simulink model "smart_watering_system_arduino"  (R2018b)
settings: Solver=FixedStepAuto  StartTime=0.0  StopTime=inf  RelTol=1e-3  EnableMultiTasking=on
settings Model: ExtModeTrigDuration=2  Creator=The MathWorks, Inc.  LastModifiedBy=Andrei
settings OptimizationCC: MaxStackSize=64
settings DebuggingCC: ParameterTunabilityLossMsg=error  LibraryContextMissingDiagnostic=none
settings HardwareCC: ProdBitPerInt=16  ProdBitPerPointer=16  ProdBitPerSizeT=16  ProdBitPerPtrDiffT=16  ProdLargestAtomicFloat=None  ProdWordSize=8  ProdHWDeviceType=Atmel->AVR  UseEmbeddedCoderFeatures=off  UseSimulinkCoderFeatures=off
settings SFSimCC: SimUseLocalCustomCode=off
settings RTWCC: SystemTargetFile=ert.tlc  HardwareBoard=Arduino Mega 2560  TemplateMakefile=ert_default_tmf  GenerateReport=on  RTWUseLocalCustomCode=off  Toolchain=Arduino AVR  BuildConfiguration=Faster Runs  LaunchReport=on
settings CodeAppCC: ForceParamTrailComments=on  OperatorAnnotations=on  StateflowObjectComments=on  MATLABSourceComments=on
settings ERTTargetCC: ERTCustomFileBanners=off  SupportContinuousTime=on  SupportNonInlinedSFcns=on  RemoveResetFunc=off  SupportVariableSizeSignals=on  ModelStepFunctionPrototypeControlCompliant=off

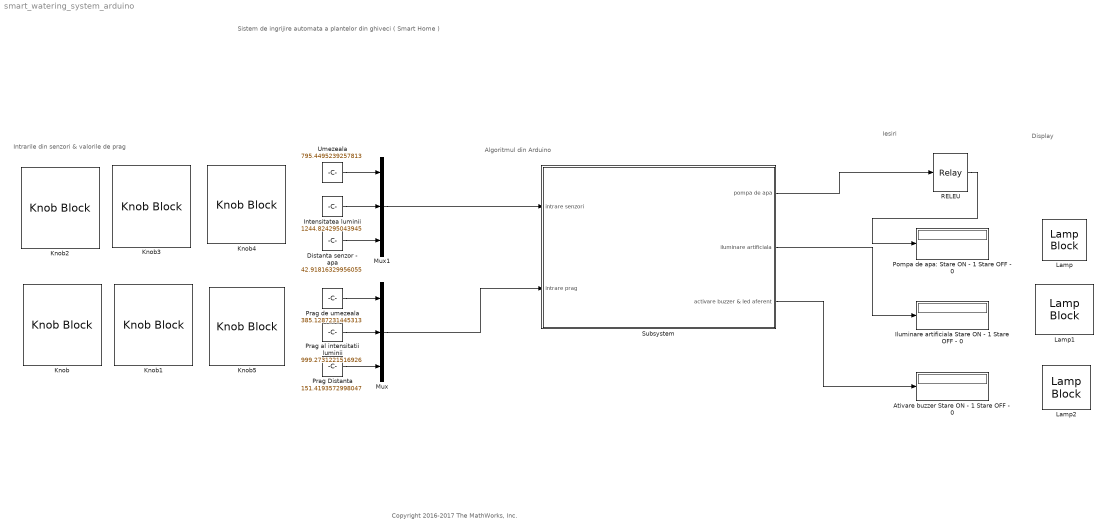
== system smart_watering_system_arduino ==
  note: Display
  note: Sistem de ingrijire automata a plantelor din ghiveci ( Smart Home )
  note: Intrarile din senzori & valorile de prag
  note: Algoritmul din Arduino
  note: Copyright 2016-2017 The MathWorks, Inc.
  note: Iesiri
  " Prag de umezeala" : Constant  Value=385.1287231445313  OutDataTypeStr=uint16
  Ativare buzzer Stare ON - 1 Stare OFF - 0 : Display
  "Distanta senzor - apa " : Constant  Value=42.91816329956055  OutDataTypeStr=uint16
  Iluminare artificiala Stare ON - 1 Stare OFF - 0 : Display
  "Intensitatea luminii " : Constant  Value=1244.824295043945  OutDataTypeStr=uint16
  Knob : KnobBlock  WebBlockId=46  ScaleMin=100  ScaleMax=700
  Knob1 : KnobBlock  WebBlockId=47  ScaleMin=500  ScaleMax=1500
  Knob2 : KnobBlock  WebBlockId=48  ScaleMax=900
  Knob3 : KnobBlock  WebBlockId=49  ScaleMax=1500
  Knob4 : KnobBlock  WebBlockId=93  ScaleMax=300
  Knob5 : KnobBlock  WebBlockId=96  ScaleMax=300
  Lamp : LampBlock  WebBlockId=91
  Lamp1 : LampBlock  WebBlockId=92
  Lamp2 : LampBlock  WebBlockId=109
  Mux : Mux  Inputs=3
  Mux1 : Mux  Inputs=3
  Pompa de apa: Stare ON - 1 Stare OFF - 0 : Display
      settings: Format=decimal (Stored Integer)
  Prag Distanta : Constant  Value=151.4193572998047  OutDataTypeStr=uint16
  Prag al intensitatii luminii : Constant  Value=999.2731221516926  OutDataTypeStr=uint16
  "RELEU " : Relay  OnSwitchValue=0.5  OffSwitchValue=0.5
  Subsystem : Subsystem
  Umezeala : Constant  Value=795.4495239257813  OutDataTypeStr=uint16
  wires:
  "Intensitatea luminii "/1 -> Mux1/2
  Subsystem/2("iluminare artificiala ") -> Iluminare artificiala Stare ON - 1 Stare OFF - 0/1
  Subsystem/1(pompa de apa) -> "RELEU "/1
  Prag al intensitatii luminii/1 -> Mux/2
  " Prag de umezeala"/1 -> Mux/1
  Umezeala/1 -> Mux1/1
  "RELEU "/1 -> Pompa de apa: Stare ON - 1 Stare OFF - 0/1
  Prag Distanta/1 -> Mux/3
  "Distanta senzor - apa "/1 -> Mux1/3
  Mux1/1 -> Subsystem/1(intrare senzori)
  Mux/1 -> Subsystem/2(intrare prag)
  Subsystem/3(activare buzzer & led aferent) -> Ativare buzzer Stare ON - 1 Stare OFF - 0/1

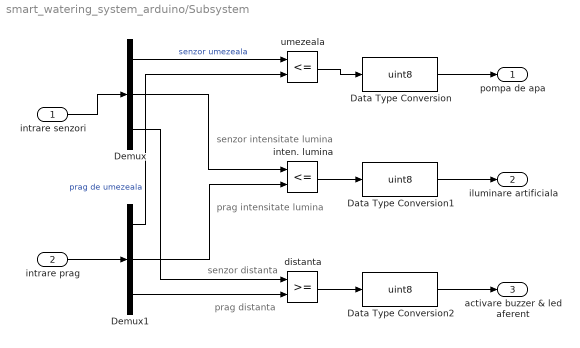
== system smart_watering_system_arduino/Subsystem ==
  note: prag intensitate lumina
  note: senzor intensitate lumina
  note: prag distanta
  note: senzor distanta
  intrare senzori : Inport
  intrare prag : Inport  Port=2
  Data Type Conversion : DataTypeConversion  OutDataTypeStr=uint8
  Data Type Conversion1 : DataTypeConversion  OutDataTypeStr=uint8
  Data Type Conversion2 : DataTypeConversion  OutDataTypeStr=uint8
  Demux : Demux  Outputs=3
  Demux1 : Demux  Outputs=3
  distanta : RelationalOperator  OutDataTypeStr=boolean  RndMeth=Simplest
  "inten. lumina " : RelationalOperator  Operator=<=  OutDataTypeStr=boolean  RndMeth=Simplest
  "umezeala " : RelationalOperator  Operator=<=  OutDataTypeStr=boolean  RndMeth=Simplest
  pompa de apa : Outport
  "iluminare artificiala " : Outport  Port=2
  activare buzzer & led aferent : Outport  Port=3
  wires:
  intrare senzori/1 -> Demux/1
  intrare prag/1 -> Demux1/1
  Demux/1 -> "umezeala "/1  "senzor umezeala"
  Demux1/1 -> "umezeala "/2  "prag de umezeala"
  Demux/2 -> "inten. lumina "/1
  Demux1/2 -> "inten. lumina "/2
  "umezeala "/1 -> Data Type Conversion/1
  Data Type Conversion/1 -> pompa de apa/1
  "inten. lumina "/1 -> Data Type Conversion1/1
  Data Type Conversion1/1 -> "iluminare artificiala "/1
  distanta/1 -> Data Type Conversion2/1
  Data Type Conversion2/1 -> activare buzzer & led aferent/1
  Demux/3 -> distanta/1
  Demux1/3 -> distanta/2
